simulink model "HW5sim"  (R2021a)
settings: Solver=VariableStepAuto  StartTime=0.0  StopTime=10  MaxStep=1e-4  RelTol=1e-3
undefined symbols (not defined in the file): bp, btheta, bz, Jp, Kistheta, Kisz, Kstheta, Ksz, Ktheta, L, theta_s_freq, theta_s_mag, velocity_command_enable, z_s_freq, z_s_mag
settings Model: Creator=LabUser  LastModifiedBy=LabUser

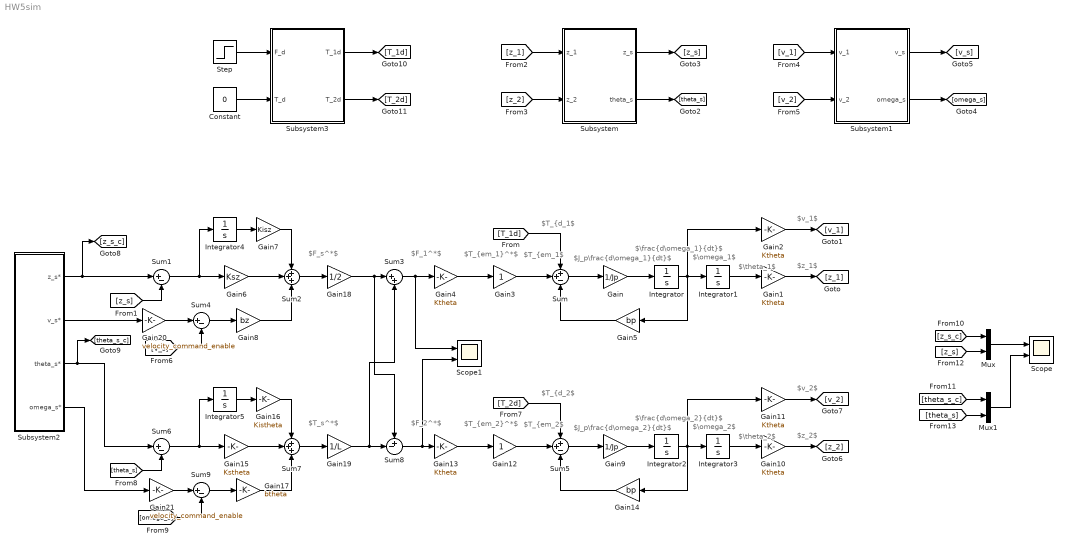
== system HW5sim ==
  note: $T_{em_1}^*$
  note: $T_{d_1$
  note: $T_{em_1$
  note: $\theta_1$
  note: $\omega_1$
  note: $z_1$
  note: $v_1$
  note: $\frac{d\omega_1}{dt}$
  note: $J_p\frac{d\omega_1}{dt}$
  note: $F_s^*$
  note: $F_1^*$
  note: $T_{d_2$
  note: $T_s^*$
  note: $v_2$
  note: $T_{em_2$
  note: $z_2$
  note: $J_p\frac{d\omega_2}{dt}$
  note: $\omega_2$
  note: $F_2^*$
  note: $\frac{d\omega_2}{dt}$
  note: $\theta_2$
  note: $T_{em_2}^*$
  Constant : Constant  Value=0
  Gain : Gain  Gain=1/Jp
  Gain{1..2,4,10..11,13} (6 alike) : Gain  Gain=Ktheta
  Gain12 : Gain
  Gain14 : Gain  Gain=bp
  Gain15 : Gain  Gain=Kstheta
  Gain16 : Gain  Gain=Kistheta
  Gain17 : Gain  Gain=btheta
  Gain18 : Gain  Gain=1/2
  Gain19 : Gain  Gain=1/L
  Gain20 : Gain  Gain=velocity_command_enable
  Gain21 : Gain  Gain=velocity_command_enable
  Gain3 : Gain
  Gain5 : Gain  Gain=bp
  Gain6 : Gain  Gain=Ksz
  Gain7 : Gain  Gain=Kisz
  Gain8 : Gain  Gain=bz
  Gain9 : Gain  Gain=1/Jp
  Integrator{,1..5} (6 alike) : Integrator
  Mux : Mux  Inputs=2
  Mux1 : Mux  Inputs=2
  Scope : Scope  NumInputPorts=2
  Scope1 : Scope  NumInputPorts=2
  Step : Step  After=1000  SampleTime=0
  Subsystem : Subsystem
  Subsystem1 : Subsystem
  Subsystem2 : Subsystem
  Subsystem3 : Subsystem
  Sum : Sum  Inputs=++-
  Sum{1,4,6,9} (4 alike) : Sum  Inputs=|+-
  Sum2 : Sum  Inputs=+++
  Sum3 : Sum  Inputs=|++
  Sum5 : Sum  Inputs=++-
  Sum7 : Sum  Inputs=+++
  Sum8 : Sum  Inputs=+-|
  wires:
  Sum/1 -> Gain/1
  Gain/1 -> Integrator/1
  Integrator/1 -> Gain5/1, Gain2/1, Integrator1/1
  Integrator1/1 -> Gain1/1
  Gain1/1 -> [z_1]
  Gain2/1 -> [v_1]
  [T_1d] -> Sum/1
  Gain3/1 -> Sum/2
  Gain4/1 -> Gain3/1
  Gain5/1 -> Sum/3
  Sum3/1 -> Scope1/1, Gain4/1
  Gain6/1 -> Sum2/2
  Gain7/1 -> Sum2/1
  Sum1/1 -> Integrator4/1, Gain6/1
  Sum4/1 -> Gain8/1
  Gain8/1 -> Sum2/3
  [z_s] -> Sum1/2
  [z_1] -> Subsystem/1(z_1)
  [z_2] -> Subsystem/2(z_2)
  Subsystem/1(z_s) -> [z_s]
  Subsystem/2(theta_s) -> [theta_s]
  Subsystem1/2(omega_s) -> [omega_s]
  Subsystem1/1(v_s) -> [v_s]
  [v_1] -> Subsystem1/1(v_1)
  [v_2] -> Subsystem1/2(v_2)
  [v_s] -> Sum4/2
  Subsystem2/1(z_s*) -> [z_s_c], Sum1/1
  [omega_s] -> Sum9/2
  Sum8/1 -> Scope1/2, Gain13/1
  Gain16/1 -> Sum7/1
  Gain15/1 -> Sum7/2
  Gain14/1 -> Sum5/3
  Gain13/1 -> Gain12/1
  Gain10/1 -> [z_2]
  Gain11/1 -> [v_2]
  Sum9/1 -> Gain17/1
  [T_2d] -> Sum5/1
  Gain9/1 -> Integrator2/1
  Gain17/1 -> Sum7/3
  Sum5/1 -> Gain9/1
  Integrator3/1 -> Gain10/1
  [theta_s] -> Sum6/2
  Gain12/1 -> Sum5/2
  Integrator2/1 -> Gain14/1, Gain11/1, Integrator3/1
  Sum6/1 -> Integrator5/1, Gain15/1
  Subsystem2/3(theta_s*) -> [theta_s_c], Sum6/1
  Sum2/1 -> Gain18/1
  Gain18/1 -> Sum8/1, Sum3/1
  Sum7/1 -> Gain19/1
  Gain19/1 -> Sum8/2, Sum3/2
  [z_s_c] -> Mux/1
  [z_s] -> Mux/2
  [theta_s_c] -> Mux1/1
  [theta_s] -> Mux1/2
  Mux/1 -> Scope/1
  Mux1/1 -> Scope/2
  Subsystem3/1(T_1d) -> [T_1d]
  Subsystem3/2(T_2d) -> [T_2d]
  Constant/1 -> Subsystem3/2(T_d)
  Step/1 -> Subsystem3/1(F_d)
  Integrator4/1 -> Gain7/1
  Integrator5/1 -> Gain16/1
  Subsystem2/2(v_s*) -> Gain20/1
  Subsystem2/4(omega_s*) -> Gain21/1
  Gain20/1 -> Sum4/1
  Gain21/1 -> Sum9/1

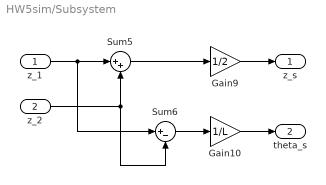
== system HW5sim/Subsystem ==
  z_1 : Inport
  z_2 : Inport  Port=2
  Gain10 : Gain  Gain=1/L
  Gain9 : Gain  Gain=1/2
  Sum5 : Sum  Inputs=|++
  Sum6 : Sum  Inputs=|+-
  z_s : Outport
  theta_s : Outport  Port=2
  wires:
  z_1/1 -> Sum6/1, Sum5/1
  Sum5/1 -> Gain9/1
  Gain10/1 -> theta_s/1
  Sum6/1 -> Gain10/1
  z_2/1 -> Sum6/2, Sum5/2
  Gain9/1 -> z_s/1

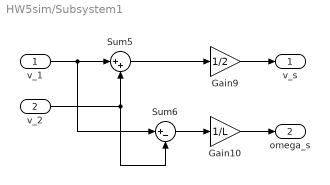
== system HW5sim/Subsystem1 ==
  v_1 : Inport
  v_2 : Inport  Port=2
  Gain10 : Gain  Gain=1/L
  Gain9 : Gain  Gain=1/2
  Sum5 : Sum  Inputs=|++
  Sum6 : Sum  Inputs=|+-
  v_s : Outport
  omega_s : Outport  Port=2
  wires:
  v_1/1 -> Sum6/1, Sum5/1
  Sum5/1 -> Gain9/1
  Gain10/1 -> omega_s/1
  Sum6/1 -> Gain10/1
  v_2/1 -> Sum6/2, Sum5/2
  Gain9/1 -> v_s/1

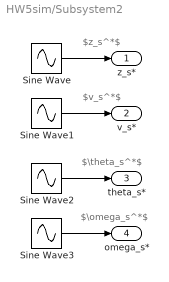
== system HW5sim/Subsystem2 ==
  note: $z_s^*$
  note: $v_s^*$
  note: $\theta_s^*$
  note: $\omega_s^*$
  Sine Wave : Sin  Amplitude=z_s_mag  Frequency=2*pi*z_s_freq  SampleTime=0
  Sine Wave1 : Sin  Amplitude=z_s_mag*2*pi*z_s_freq  Frequency=2*pi*z_s_freq  Phase=pi/2  SampleTime=0
  Sine Wave2 : Sin  Amplitude=theta_s_mag  Frequency=2*pi*theta_s_freq  SampleTime=0
  Sine Wave3 : Sin  Amplitude=theta_s_mag*2*pi*theta_s_freq  Frequency=2*pi*theta_s_freq  Phase=pi/2  SampleTime=0
  z_s* : Outport
  v_s* : Outport  Port=2
  theta_s* : Outport  Port=3
  omega_s* : Outport  Port=4
  wires:
  Sine Wave2/1 -> theta_s*/1
  Sine Wave/1 -> z_s*/1
  Sine Wave1/1 -> v_s*/1
  Sine Wave3/1 -> omega_s*/1

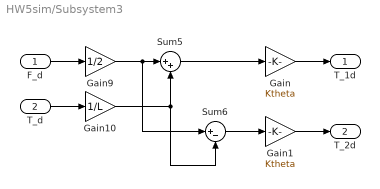
== system HW5sim/Subsystem3 ==
  F_d : Inport
  T_d : Inport  Port=2
  Gain : Gain  Gain=Ktheta
  Gain1 : Gain  Gain=Ktheta
  Gain10 : Gain  Gain=1/L
  Gain9 : Gain  Gain=1/2
  Sum5 : Sum  Inputs=|++
  Sum6 : Sum  Inputs=|+-
  T_1d : Outport
  T_2d : Outport  Port=2
  wires:
  Sum5/1 -> Gain/1
  T_d/1 -> Gain10/1
  Sum6/1 -> Gain1/1
  F_d/1 -> Gain9/1
  Gain9/1 -> Sum5/1, Sum6/1
  Gain10/1 -> Sum5/2, Sum6/2
  Gain1/1 -> T_2d/1
  Gain/1 -> T_1d/1
